simulink model "QPC"  (R2017b)
settings: Solver=VariableStepAuto  StartTime=0.0  StopTime=10.0  RelTol=1e-3
libraries: commrandsrc3 x15, commutil2 x13
settings Model: Creator=Alexander  LastModifiedBy=a.egorov

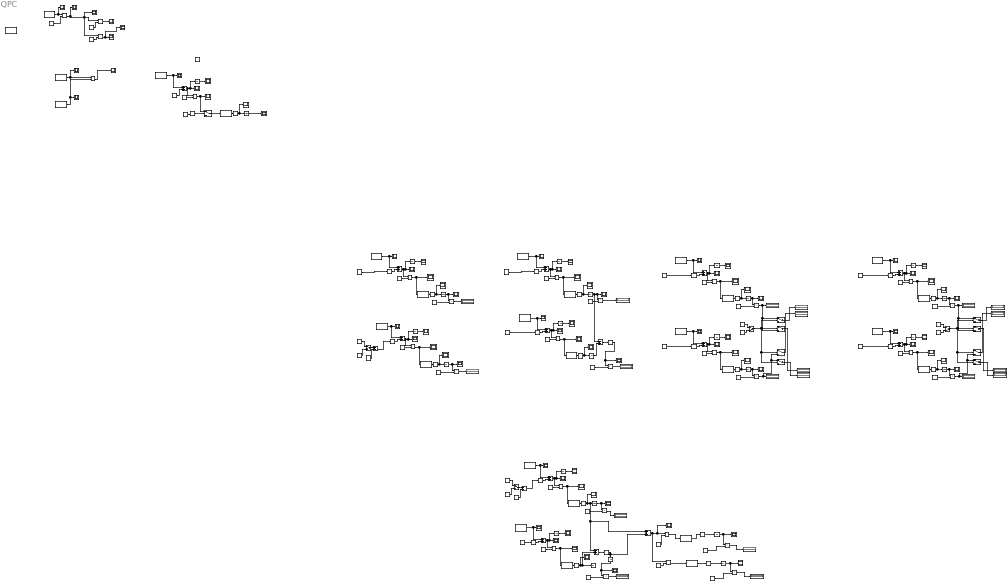
== system QPC ==
  note: ХЕЛЛОУ ВОРЛД
  note: NOT gate
  note: Вход
  note: Вход 1
  note: СNOT gate
  note: H gate
  note: Вход 1
  note: Вход 2
  note: Вход
  note: SWAP
  note: Вход
  note: Вход
  note: ПОКА CSWAP НЕ РАБОТАЕТ
  note: Вход
  note: 2 кубит
  note: Вход 1
  note: Вход 2
  note: Вход 1
  note: 1 кубит
  Abs{,1..24} (25 alike) : Abs
  Add{,1..3,5,7..11,13,15} (12 alike) : Sum
  Add12 : Sum  Inputs=+-
  Add14 : Sum  Inputs=-+
  Add4 : Sum  Inputs=-+
  Add6 : Sum  Inputs=+-
  Bit to Integer Converter{,1..12} (13 alike) : commutil2/Bit to Integer Converter  nbits=1  bitOrder=MSB first  signedOutputValues=Signed  outDtype=Inherit via internal rule  outDtypeSigned=double
  Constant{,1,15,28,34,38} (6 alike) : Constant
  Constant{2,7..8,10,12,21,25,29,32,35,40,43} (12 alike) : Constant  Value=100
  Constant{6,11,16..20,22..23,26,30,39,42,46..47} (15 alike) : Constant  Value=10
  Constant{4..5,13,27,33,36,41,45} (8 alike) : Constant  Value=0
  Constant14 : Constant  Value=50
  Constant24 : Constant  Value=40
  Constant3 : Constant  Value=20
  Constant31 : Constant  Value=40
  Constant37 : Constant  Value=50
  Constant44 : Constant  Value=2
  Constant9 : Constant  Value=30
  Display{,1..19} (20 alike) : Display
  Divide : Product  Inputs=*/
  Divide1 : Product  Inputs=*/
  Integrator{,1..24} (25 alike) : Integrator
  Manual Switch : ManualSwitch
  Manual Switch1 : ManualSwitch  CurrentSetting=0
  Manual Switch2 : ManualSwitch  CurrentSetting=0
  Manual Switch3 : ManualSwitch
  Product{,1..11} (12 alike) : Product
  Random Integer Generator : commrandsrc3/Random Integer Generator  SetSize=20  SeedSource=Auto  Seed=0  SampleTime=0.01  SamplesPerFrame=1  OutputDataType=uint32  SimulateUsing=Interpreted execution
  Random Integer Generator1 : commrandsrc3/Random Integer Generator  SetSize=21  SeedSource=Auto  Seed=0  SampleTime=0.01  SamplesPerFrame=1  OutputDataType=single  SimulateUsing=Interpreted execution
  Random Integer Generator{4..11,13} (9 alike) : commrandsrc3/Random Integer Generator  SetSize=101  SeedSource=Auto  Seed=0  SampleTime=0.01  SamplesPerFrame=1  OutputDataType=single  SimulateUsing=Interpreted execution
  Random Integer Generator12 : commrandsrc3/Random Integer Generator  SetSize=101  SeedSource=Auto  Seed=0  SampleTime=0.001  SamplesPerFrame=1  OutputDataType=single  SimulateUsing=Interpreted execution
  Random Integer Generator14 : commrandsrc3/Random Integer Generator  SetSize=101  SeedSource=Auto  Seed=0  SampleTime=0.001  SamplesPerFrame=1  OutputDataType=single  SimulateUsing=Interpreted execution
  Random Integer Generator2 : commrandsrc3/Random Integer Generator  SetSize=2  SeedSource=Auto  Seed=0  SampleTime=0.01  SamplesPerFrame=1  OutputDataType=single  SimulateUsing=Interpreted execution
  Random Integer Generator3 : commrandsrc3/Random Integer Generator  SetSize=2  SeedSource=Auto  Seed=0  SampleTime=0.01  SamplesPerFrame=1  OutputDataType=single  SimulateUsing=Interpreted execution
  Relational Operator{,1..4} (5 alike) : RelationalOperator  Operator===  OutDataTypeStr=boolean  RndMeth=Simplest
  Relational Operator{5..14} (10 alike) : RelationalOperator  OutDataTypeStr=boolean  RndMeth=Simplest
  Relational Operator15 : RelationalOperator  Operator===  OutDataTypeStr=boolean  ZeroCross=off  RndMeth=Simplest
  Relational Operator16 : RelationalOperator  Operator===  OutDataTypeStr=boolean  ZeroCross=off  RndMeth=Simplest
  Scope{,1..76} (77 alike) : Scope
  Switch : Switch  Criteria=u2 > Threshold
  Switch{1..8} (8 alike) : Switch  Criteria=u2 ~= 0
  Чекаем что достаточно случайно вообще : Scope
  wires:
  Constant1/1 -> Relational Operator/2
  Relational Operator/1 -> Scope/1
  Constant3/1 -> Divide/2
  Random Integer Generator1/1 -> Scope3/1, Divide/1
  Divide/1 -> Relational Operator1/1, Scope2/1, Relational Operator/1, Scope1/1
  Constant4/1 -> Relational Operator1/2
  Relational Operator1/1 -> Scope5/1, Scope4/1
  Random Integer Generator2/1 -> Scope6/1, Relational Operator2/1
  Random Integer Generator3/1 -> Relational Operator2/2, Scope7/1
  Relational Operator2/1 -> Чекаем что достаточно случайно вообще/1
  Random Integer Generator4/1 -> Add/1, Scope8/1
  Constant/1 -> Add/2
  Add/1 -> Relational Operator3/1, Integrator1/1, Scope9/1
  Constant2/1 -> Relational Operator3/2
  Relational Operator3/1 -> Switch/1, Scope10/1
  Integrator/1 -> Scope11/1
  Bit to Integer Converter/1 -> Abs/1
  Abs/1 -> Integrator/1, Scope12/1
  Integrator1/1 -> Scope13/1
  Constant5/1 -> Relational Operator4/2
  Abs1/1 -> Integrator2/1, Scope16/1
  Constant7/1 -> Relational Operator5/2
  Bit to Integer Converter1/1 -> Abs1/1
  Relational Operator5/1 -> Bit to Integer Converter1/1, Scope14/1
  Integrator3/1 -> Scope17/1
  Random Integer Generator5/1 -> Add1/1, Scope18/1
  Add1/1 -> Relational Operator5/1, Integrator3/1, Scope19/1
  Switch/1 -> Bit to Integer Converter/1
  Relational Operator4/1 -> Switch/2
  Constant6/1 -> Abs2/1
  Abs2/1 -> Add1/2
  Abs4/1 -> Add3/2
  Constant9/1 -> Abs4/1
  Add3/1 -> Relational Operator6/1, Integrator5/1, Scope25/1
  Integrator5/1 -> Scope23/1
  Integrator4/1 -> Add4/1, Product/1, Scope21/1
  Relational Operator6/1 -> Bit to Integer Converter2/1, Scope20/1
  Abs3/1 -> Integrator4/1, Scope22/1
  Random Integer Generator6/1 -> Add3/1, Scope24/1
  Constant10/1 -> Relational Operator6/2
  Bit to Integer Converter2/1 -> Abs3/1
  Constant12/1 -> Relational Operator7/2
  Bit to Integer Converter3/1 -> Abs5/1
  Integrator7/1 -> Scope29/1
  Relational Operator7/1 -> Bit to Integer Converter3/1, Scope26/1
  Abs5/1 -> Integrator6/1, Scope28/1
  Abs6/1 -> Add5/2
  Add5/1 -> Relational Operator7/1, Integrator7/1, Scope31/1
  Random Integer Generator7/1 -> Add5/1, Scope30/1
  Constant13/1 -> Manual Switch/1
  Constant15/1 -> Manual Switch/2
  Manual Switch/1 -> Add6/1
  Constant14/1 -> Add6/2
  Add6/1 -> Abs6/1
  Constant16/1 -> Product/2
  Product/1 -> Display/1
  Constant17/1 -> Product1/2
  Product1/1 -> Display1/1
  Integrator2/1 -> Product1/1, Scope15/1
  Constant18/1 -> Product2/2
  Product2/1 -> Display2/1
  Integrator6/1 -> Product2/1, Scope27/1
  Abs8/1 -> Add7/2
  Constant20/1 -> Abs8/1
  Add7/1 -> Relational Operator8/1, Integrator9/1, Scope37/1
  Integrator9/1 -> Scope35/1
  Integrator8/1 -> Product3/1, Scope33/1
  Relational Operator8/1 -> Bit to Integer Converter4/1, Scope32/1
  Abs7/1 -> Integrator8/1, Scope34/1
  Random Integer Generator8/1 -> Add7/1, Scope36/1
  Constant21/1 -> Relational Operator8/2
  Product3/1 -> Switch4/3, Switch1/1, Display3/1
  Constant19/1 -> Product3/2
  Bit to Integer Converter4/1 -> Abs7/1
  Abs10/1 -> Add9/2
  Constant24/1 -> Abs10/1
  Add9/1 -> Relational Operator9/1, Integrator11/1, Scope43/1
  Integrator11/1 -> Scope41/1
  Integrator10/1 -> Product4/1, Scope39/1
  Relational Operator9/1 -> Bit to Integer Converter5/1, Scope38/1
  Abs9/1 -> Integrator10/1, Scope40/1
  Random Integer Generator9/1 -> Add9/1, Scope42/1
  Constant25/1 -> Relational Operator9/2
  Product4/1 -> Switch3/3, Switch2/1, Display4/1
  Constant23/1 -> Product4/2
  Bit to Integer Converter5/1 -> Abs9/1
  Switch1/1 -> Display5/1
  Switch2/1 -> Display6/1
  Constant28/1 -> Manual Switch1/1
  Constant27/1 -> Manual Switch1/2
  Manual Switch1/1 -> Switch4/2, Switch3/2, Switch2/2, Switch1/2
  Switch4/1 -> Display7/1
  Switch3/1 -> Display8/1
  Constant26/1 -> Abs13/1
  Switch8/1 -> Display13/1
  Constant33/1 -> Manual Switch2/2
  Add8/1 -> Relational Operator10/1, Integrator15/1, Scope49/1
  Abs13/1 -> Add8/2
  Switch7/1 -> Display14/1
  Bit to Integer Converter6/1 -> Abs12/1
  Product5/1 -> Switch8/3, Switch5/1, Display9/1
  Constant29/1 -> Relational Operator10/2
  Abs12/1 -> Integrator14/1, Scope46/1
  Constant34/1 -> Manual Switch2/1
  Relational Operator10/1 -> Bit to Integer Converter6/1, Scope44/1
  Product6/1 -> Switch7/3, Switch6/1, Display10/1
  Random Integer Generator11/1 -> Add10/1, Scope54/1
  Random Integer Generator10/1 -> Add8/1, Scope48/1
  Constant22/1 -> Product5/2
  Constant31/1 -> Abs11/1
  Relational Operator11/1 -> Bit to Integer Converter7/1, Scope50/1
  Constant30/1 -> Product6/2
  Integrator13/1 -> Scope53/1
  Switch6/1 -> Display12/1
  Abs14/1 -> Integrator12/1, Scope52/1
  Add10/1 -> Relational Operator11/1, Integrator13/1, Scope55/1
  Integrator15/1 -> Scope47/1
  Manual Switch2/1 -> Switch8/2, Switch7/2, Switch6/2, Switch5/2
  Abs11/1 -> Add10/2
  Integrator14/1 -> Product5/1, Scope45/1
  Bit to Integer Converter7/1 -> Abs14/1
  Integrator12/1 -> Product6/1, Scope51/1
  Constant32/1 -> Relational Operator11/2
  Switch5/1 -> Display11/1
  Manual Switch3/1 -> Add12/1
  Bit to Integer Converter8/1 -> Abs15/1
  Relational Operator12/1 -> Bit to Integer Converter8/1, Scope56/1
  Integrator17/1 -> Scope59/1
  Abs16/1 -> Add11/2
  Abs15/1 -> Add15/1, Add14/1, Integrator16/1, Scope58/1
  Random Integer Generator12/1 -> Add11/1, Scope60/1
  Constant37/1 -> Add12/2
  Constant38/1 -> Manual Switch3/2
  Constant36/1 -> Manual Switch3/1
  Add11/1 -> Relational Operator12/1, Integrator17/1, Scope61/1
  Constant39/1 -> Product7/2
  Add12/1 -> Abs16/1
  Product7/1 -> Display15/1
  Constant35/1 -> Relational Operator12/2
  Constant42/1 -> Product8/2
  Product8/1 -> Display16/1
  Constant40/1 -> Relational Operator13/2
  Bit to Integer Converter9/1 -> Abs17/1
  Integrator19/1 -> Scope65/1
  Relational Operator13/1 -> Bit to Integer Converter9/1, Scope62/1
  Abs17/1 -> Integrator18/1, Scope64/1
  Abs18/1 -> Add13/2
  Add13/1 -> Relational Operator13/1, Integrator19/1, Scope67/1
  Random Integer Generator13/1 -> Add13/1, Scope66/1
  Constant43/1 -> Abs18/1
  Add4/1 -> Abs19/1
  Integrator18/1 -> Add4/2
  Abs19/1 -> Scope63/1, Product8/1
  Random Integer Generator14/1 -> Add2/1, Scope72/1
  Relational Operator14/1 -> Bit to Integer Converter10/1, Scope68/1
  Abs20/1 -> Integrator20/1, Add14/2, Scope70/1
  Abs21/1 -> Add2/2
  Constant11/1 -> Product9/2
  Bit to Integer Converter10/1 -> Abs20/1
  Constant8/1 -> Relational Operator14/2
  Abs22/1 -> Add15/2, Integrator22/1
  Integrator21/1 -> Scope71/1
  Add2/1 -> Relational Operator14/1, Integrator21/1, Scope73/1
  Product9/1 -> Display17/1
  Integrator16/1 -> Product7/1, Scope57/1
  Add14/1 -> Abs22/1
  Constant41/1 -> Abs21/1
  Add15/1 -> Relational Operator16/1, Scope75/1, Relational Operator15/1
  Constant44/1 -> Relational Operator15/2
  Relational Operator15/1 -> Bit to Integer Converter11/1
  Integrator22/1 -> Scope69/1, Product9/1
  Integrator23/1 -> Product10/1, Scope74/1
  Abs23/1 -> Integrator23/1
  Bit to Integer Converter11/1 -> Abs23/1
  Constant45/1 -> Relational Operator16/2
  Abs24/1 -> Integrator24/1
  Bit to Integer Converter12/1 -> Abs24/1
  Integrator24/1 -> Product11/1, Scope76/1
  Relational Operator16/1 -> Bit to Integer Converter12/1
  Constant46/1 -> Product10/2
  Product10/1 -> Display19/1
  Constant47/1 -> Product11/2
  Product11/1 -> Display18/1
